simulink model "IDENTIFICACION_ARX_ARMAX"  (R2013a)
settings: Solver=ode5  SolverMode=SingleTasking  StartTime=0.0  StopTime=130  RelTol=1e-3
values from neighbouring files (symbols this model uses):
  lambda = 1    [generar_prbs.m]    (also in parametros_ident.m = 0.995)
undefined symbols (not defined in the file or in its folder): National_Instruments, PCI
libraries: rtwinlib x2
settings Model: SimulationMode=external  ExtModeTrigDuration=100000  Creator=n221  LastModifiedBy=u_labelectro
settings DataIOCC: SignalLoggingSaveFormat=ModelDataLogs
settings OptimizationCC: BlockReduction=off  BooleanDataType=off
settings DebuggingCC: SaveWithParameterizedLinksMsg=none  SignalResolutionControl=TryResolveAllWithWarning  SolverPrmCheckMsg=none  MultiTaskDSMMsg=warning  MultiTaskCondExecSysMsg=none  StrictBusMsg=None
settings HardwareCC: ProdIntDivRoundTo=Zero  ProdEndianess=LittleEndian  ProdHWDeviceType=Generic->32-bit x86 compatible  TargetIntDivRoundTo=Zero  TargetEndianess=LittleEndian  TargetHWDeviceType=MATLAB Host  ProdEqTarget=off
settings RTWCC: SystemTargetFile=rtwin.tlc  TemplateMakefile=rtwin.tmf  Description=Real-Time Windows Target  ProcessScript=rtwin_make_rtw_hook  IncludeERTFirstTime=on  RTWCompilerOptimization=On
settings CodeAppCC: MaxIdLength=95
settings RTWinTargetCC: TargetLibSuffix=_rtwin.lib  TargetPreCompLibLocation=D:\Real Time\toolbox\rtw\targets\rtwin\lib\win64  CodeReplacementLibrary=ANSI_C  RTWinDir=D:/REALTI~1/toolbox/rtw/targets/rtwin  TargetArch=win64

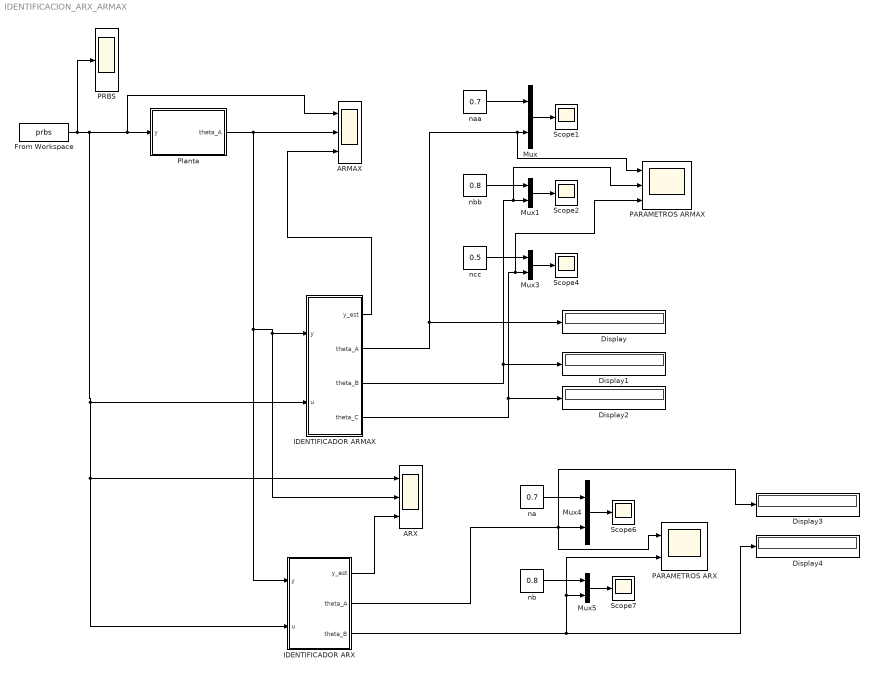
== system IDENTIFICACION_ARX_ARMAX ==
  ARMAX : Scope  NumInputPorts=3
      settings: TimeRange=130  YMin=20~42.5~45  YMax=20~70~75  SaveName=SALIDA_ARMAX  SampleInput=on  SampleTime=0.01
  ARX : Scope  NumInputPorts=3
      settings: YMin=-5~-5~-5  YMax=5~5~5  SaveName=SALIDA_ARX  SampleInput=on  SampleTime=0.01
  Display{,1..4} (5 alike) : Display
  From Workspace : FromWorkspace  VariableName=prbs  SampleTime=0.01
  IDENTIFICADOR ARMAX : Subsystem
  IDENTIFICADOR ARX : Subsystem
  Mux{,1,3..5} (5 alike) : Mux  Inputs=2
  PARAMETROS ARMAX : Scope  NumInputPorts=3
      settings: TimeRange=130  YMin=-0.99925~0.00075~0.005  YMax=-0.99475~0.00375~0.035  SaveName=PARAMETROS_ARMAX  SampleInput=on  SampleTime=0.01
  PARAMETROS ARX : Scope  NumInputPorts=2
      settings: TimeRange=600  YMin=-0.8~-5  YMax=0.8~5  SaveName=PARAMETROS_ARX  SampleInput=on  SampleTime=0.01
  PRBS : Scope
      settings: SaveName=ScopeData3  SampleInput=on  SampleTime=0.01
  Planta : Subsystem
  Scope{1..2,4,6..7} (5 alike) : Scope
      Scope1 settings: TimeRange=600  YMin=-0.8  YMax=0.8  SampleInput=on  SampleTime=0.01
      Scope2 settings: SaveName=ScopeData2  SampleInput=on  SampleTime=0.01
      Scope4 settings: SaveName=ScopeData4  SampleInput=on  SampleTime=0.01
      Scope6 settings: TimeRange=600  YMin=-0.8  YMax=0.8  SaveName=ScopeData6  SampleInput=on  SampleTime=0.01
      Scope7 settings: SaveName=ScopeData7  SampleInput=on  SampleTime=0.01
  na : Constant  Value=0.7
  "naa " : Constant  Value=0.7
  nb : Constant  Value=0.8
  nbb : Constant  Value=0.8
  ncc : Constant  Value=0.5
  wires:
  "naa "/1 -> Mux/1
  IDENTIFICADOR ARMAX/2(theta_A) -> PARAMETROS ARMAX/1, Mux/2, Display/1
  nbb/1 -> Mux1/1
  Mux1/1 -> Scope2/1
  Mux/1 -> Scope1/1
  IDENTIFICADOR ARMAX/3(theta_B) -> PARAMETROS ARMAX/2, Mux1/2, Display1/1
  IDENTIFICADOR ARMAX/4(theta_C) -> Display2/1, PARAMETROS ARMAX/3, Mux3/2
  Mux3/1 -> Scope4/1
  ncc/1 -> Mux3/1
  From Workspace/1 -> PRBS/1, ARX/1, IDENTIFICADOR ARX/2(u), IDENTIFICADOR ARMAX/2(u), Planta/1(y), ARMAX/1
  na/1 -> Mux4/1
  nb/1 -> Mux5/1
  Mux5/1 -> Scope7/1
  Mux4/1 -> Scope6/1
  IDENTIFICADOR ARX/2(theta_A) -> PARAMETROS ARX/1, Display3/1, Mux4/2
  IDENTIFICADOR ARX/3(theta_B) -> Display4/1, Mux5/2, PARAMETROS ARX/2
  IDENTIFICADOR ARMAX/1(y_est) -> ARMAX/3
  IDENTIFICADOR ARX/1(y_est) -> ARX/3
  Planta/1(theta_A) -> IDENTIFICADOR ARX/1(y), ARX/2, IDENTIFICADOR ARMAX/1(y), ARMAX/2

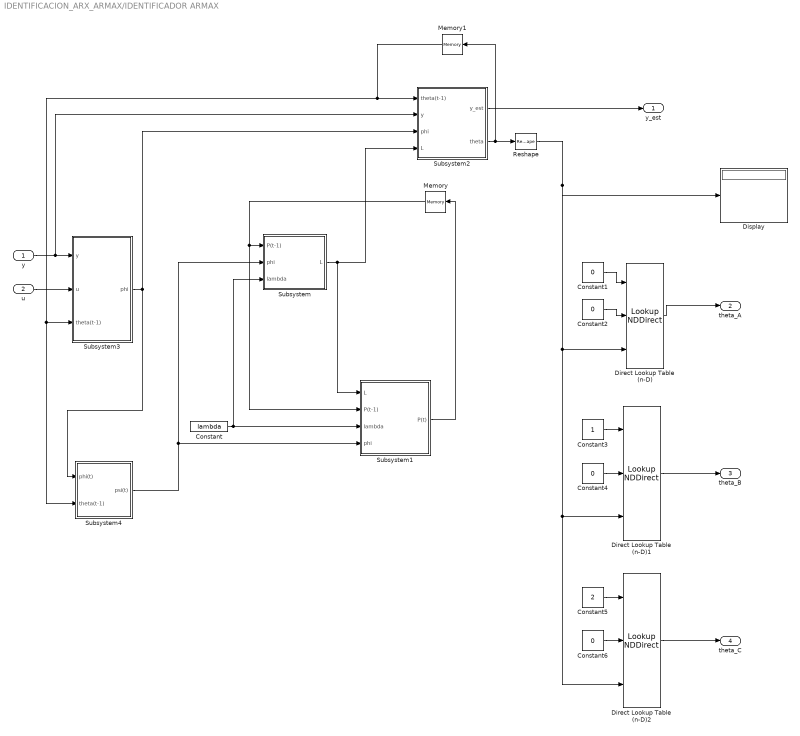
== system IDENTIFICACION_ARX_ARMAX/IDENTIFICADOR ARMAX ==
  y : Inport
  u : Inport  Port=2
  Constant : Constant  Value=lambda
  Constant{1..2,4,6} (4 alike) : Constant  Value=0
  Constant3 : Constant
  Constant5 : Constant  Value=2
  Direct Lookup Table (n-D) : LookupNDDirect  TableIsInput=on  Table=[4 5 ;16 19 ]  DiagnosticForOutOfRangeInput=Error  SampleTime=0.01
  Direct Lookup Table (n-D)1 : LookupNDDirect  TableIsInput=on  Table=[4 5 ;16 19 ]  DiagnosticForOutOfRangeInput=Error  SampleTime=0.01
  Direct Lookup Table (n-D)2 : LookupNDDirect  TableIsInput=on  Table=[4 5 ;16 19 ]  DiagnosticForOutOfRangeInput=Error  SampleTime=0.01
  Display : Display
  Memory : Memory  X0=1e6*eye(3)
  Memory1 : Memory
  Reshape : Reshape  OutputDimensionality=Column vector (2-D)
  Subsystem : Subsystem
  Subsystem1 : Subsystem
  Subsystem2 : Subsystem
  Subsystem3 : Subsystem
  Subsystem4 : Subsystem
  y_est : Outport
  theta_A : Outport  Port=2
  theta_B : Outport  Port=3
  theta_C : Outport  Port=4
  wires:
  y/1 -> Subsystem2/2(y), Subsystem3/1(y)
  Subsystem3/1(phi) -> Subsystem2/3(phi), Subsystem4/1(phi(t))
  Subsystem/1(L) -> Subsystem1/1(L), Subsystem2/4(L)
  u/1 -> Subsystem3/2(u)
  Constant/1 -> Subsystem1/3(lambda), Subsystem/3(lambda)
  Subsystem1/1(P(t)) -> Memory/1
  Memory/1 -> Subsystem1/2(P(t-1)), Subsystem/1(P(t-1))
  Subsystem2/1(y_est) -> y_est/1
  Subsystem2/2(theta) -> Reshape/1, Memory1/1
  Memory1/1 -> Subsystem4/2(theta(t-1)), Subsystem3/3(theta(t-1)), Subsystem2/1(theta(t-1))
  Constant4/1 -> Direct Lookup Table (n-D)1/2
  Constant3/1 -> Direct Lookup Table (n-D)1/1
  Constant1/1 -> Direct Lookup Table (n-D)/1
  Direct Lookup Table (n-D)/1 -> theta_A/1
  Direct Lookup Table (n-D)1/1 -> theta_B/1
  Constant2/1 -> Direct Lookup Table (n-D)/2
  Constant6/1 -> Direct Lookup Table (n-D)2/2
  Constant5/1 -> Direct Lookup Table (n-D)2/1
  Direct Lookup Table (n-D)2/1 -> theta_C/1
  Reshape/1 -> Direct Lookup Table (n-D)/3, Direct Lookup Table (n-D)2/3, Direct Lookup Table (n-D)1/3, Display/1
  Subsystem4/1(psi(t)) -> Subsystem1/4(phi), Subsystem/2(phi)

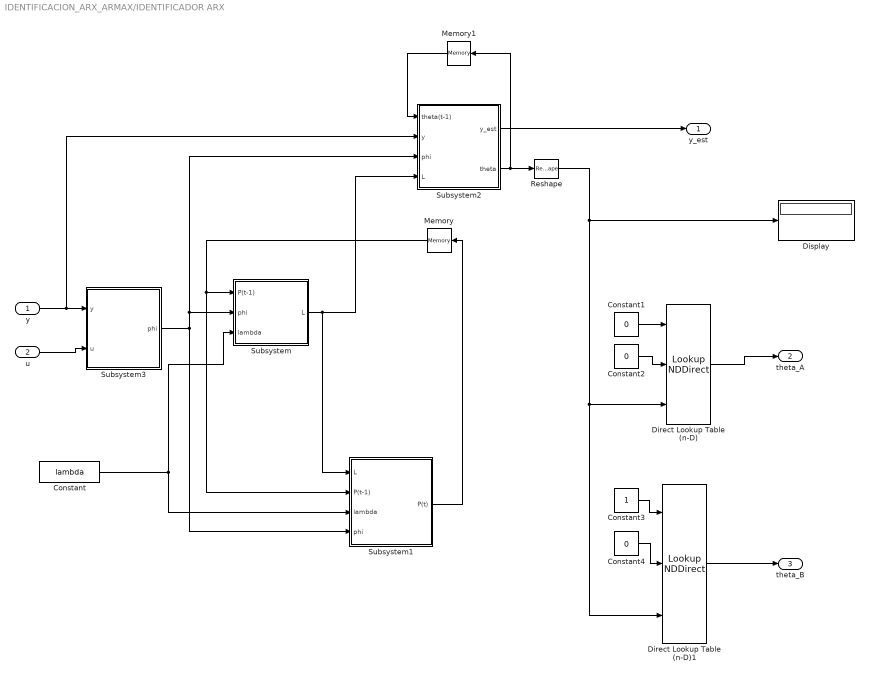
== system IDENTIFICACION_ARX_ARMAX/IDENTIFICADOR ARX ==
  y : Inport
  u : Inport  Port=2
  Constant : Constant  Value=lambda
  Constant1 : Constant  Value=0
  Constant2 : Constant  Value=0
  Constant3 : Constant
  Constant4 : Constant  Value=0
  Direct Lookup Table (n-D) : LookupNDDirect  TableIsInput=on  Table=[4 5 ;16 19 ]  DiagnosticForOutOfRangeInput=Error
  Direct Lookup Table (n-D)1 : LookupNDDirect  TableIsInput=on  Table=[4 5 ;16 19 ]  DiagnosticForOutOfRangeInput=Error
  Display : Display
  Memory : Memory  X0=1e6*eye(2)
  Memory1 : Memory
  Reshape : Reshape  OutputDimensionality=Column vector (2-D)
  Subsystem : Subsystem
  Subsystem1 : Subsystem
  Subsystem2 : Subsystem
  Subsystem3 : Subsystem
  y_est : Outport
  theta_A : Outport  Port=2
  theta_B : Outport  Port=3
  wires:
  y/1 -> Subsystem2/2(y), Subsystem3/1(y)
  Subsystem3/1(phi) -> Subsystem1/4(phi), Subsystem2/3(phi), Subsystem/2(phi)
  Subsystem/1(L) -> Subsystem1/1(L), Subsystem2/4(L)
  u/1 -> Subsystem3/2(u)
  Constant/1 -> Subsystem1/3(lambda), Subsystem/3(lambda)
  Subsystem1/1(P(t)) -> Memory/1
  Memory/1 -> Subsystem1/2(P(t-1)), Subsystem/1(P(t-1))
  Subsystem2/1(y_est) -> y_est/1
  Subsystem2/2(theta) -> Reshape/1, Memory1/1
  Memory1/1 -> Subsystem2/1(theta(t-1))
  Constant4/1 -> Direct Lookup Table (n-D)1/2
  Constant3/1 -> Direct Lookup Table (n-D)1/1
  Constant2/1 -> Direct Lookup Table (n-D)/2
  Constant1/1 -> Direct Lookup Table (n-D)/1
  Reshape/1 -> Direct Lookup Table (n-D)1/3, Direct Lookup Table (n-D)/3, Display/1
  Direct Lookup Table (n-D)/1 -> theta_A/1
  Direct Lookup Table (n-D)1/1 -> theta_B/1

== system IDENTIFICACION_ARX_ARMAX/Planta ==
  y : Inport
  Analog Input : rtwinlib/Analog Input  SampleTime=0.1  MaxMissedTicks=10  ShowMissedTicks=off  YieldWhenWaiting=off  DrvName=National_Instruments/PCI-6229  DrvAddress=4294967295  DrvOptions=[0 0 0 0 0]  Channels=1  RangeMode=1  VoltRange=1  DataType=1
      settings: AttributesFormatString=National Instruments\nPCI-6229 [auto]
  Analog Output : rtwinlib/Analog Output  SampleTime=0.1  MaxMissedTicks=10  ShowMissedTicks=off  YieldWhenWaiting=off  DrvName=National_Instruments/PCI-6229  DrvAddress=4294967295  DrvOptions=[0 0 0 0 0]  Channels=1  RangeMode=1  VoltRange=1  InitialValue=[]  FinalValue=[]
      settings: AttributesFormatString=National Instruments\nPCI-6229 [auto]
  Fcn : Fcn  Expr=0.2*u(1)-10
  Fcn1 : Fcn  Expr=25*u(1)-25
  theta_A : Outport
  wires:
  Fcn/1 -> Analog Output/1
  y/1 -> Fcn/1
  Analog Input/1 -> Fcn1/1
  Fcn1/1 -> theta_A/1

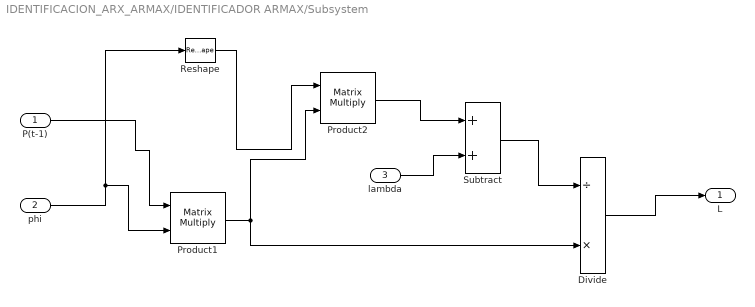
== system IDENTIFICACION_ARX_ARMAX/IDENTIFICADOR ARMAX/Subsystem ==
  P(t-1) : Inport
  phi : Inport  Port=2
  lambda : Inport  Port=3
  Divide : Product  Inputs=/*
  Product1 : Product  Multiplication=Matrix(*)  SampleTime=0.01
  Product2 : Product  Multiplication=Matrix(*)  SampleTime=0.01
  Reshape : Reshape  OutputDimensionality=Row vector (2-D)
  Subtract : Sum
  L : Outport
  wires:
  Divide/1 -> L/1
  Subtract/1 -> Divide/1
  phi/1 -> Product1/2, Reshape/1
  Reshape/1 -> Product2/1
  lambda/1 -> Subtract/2
  Product1/1 -> Divide/2, Product2/2
  P(t-1)/1 -> Product1/1
  Product2/1 -> Subtract/1

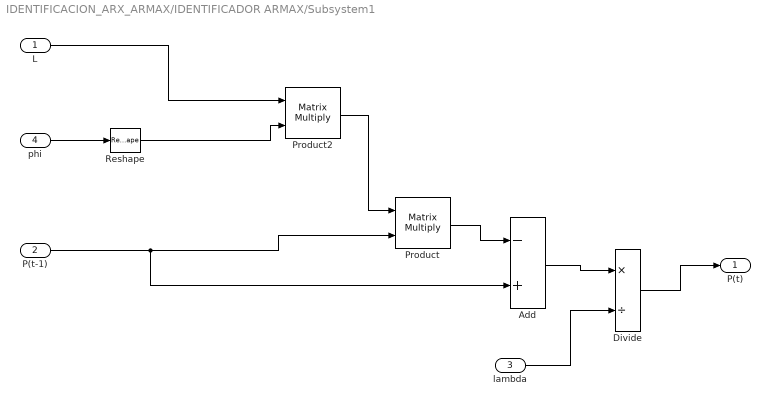
== system IDENTIFICACION_ARX_ARMAX/IDENTIFICADOR ARMAX/Subsystem1 ==
  L : Inport
  P(t-1) : Inport  Port=2
  lambda : Inport  Port=3
  phi : Inport  Port=4
  Add : Sum  Inputs=-+
  Divide : Product  Inputs=*/
  Product : Product  Multiplication=Matrix(*)  SampleTime=0.01
  Product2 : Product  Multiplication=Matrix(*)  SampleTime=0.01
  Reshape : Reshape  OutputDimensionality=Row vector (2-D)
  P(t) : Outport
  wires:
  L/1 -> Product2/1
  phi/1 -> Reshape/1
  Reshape/1 -> Product2/2
  Product2/1 -> Product/1
  P(t-1)/1 -> Product/2, Add/2
  Product/1 -> Add/1
  Add/1 -> Divide/1
  Divide/1 -> P(t)/1
  lambda/1 -> Divide/2

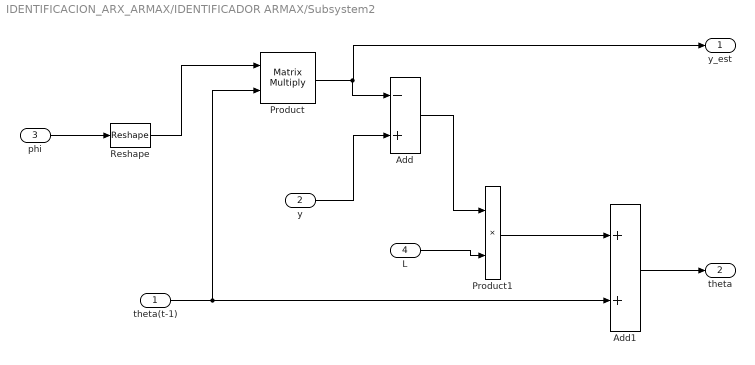
== system IDENTIFICACION_ARX_ARMAX/IDENTIFICADOR ARMAX/Subsystem2 ==
  theta(t-1) : Inport
  y : Inport  Port=2
  phi : Inport  Port=3
  L : Inport  Port=4
  Add : Sum  Inputs=-+
  Add1 : Sum
  Product : Product  Multiplication=Matrix(*)  SampleTime=0.01
  Product1 : Product
  Reshape : Reshape  OutputDimensionality=Row vector (2-D)
  y_est : Outport
  theta : Outport  Port=2
  wires:
  Product/1 -> Add/1, y_est/1
  y/1 -> Add/2
  L/1 -> Product1/2
  Add/1 -> Product1/1
  Product1/1 -> Add1/1
  Add1/1 -> theta/1
  theta(t-1)/1 -> Product/2, Add1/2
  Reshape/1 -> Product/1
  phi/1 -> Reshape/1

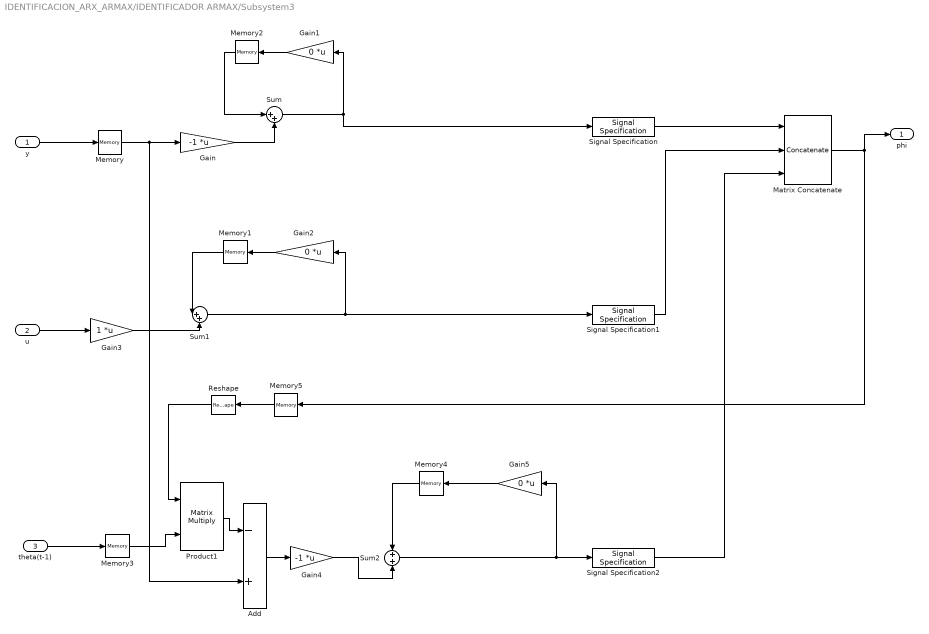
== system IDENTIFICACION_ARX_ARMAX/IDENTIFICADOR ARMAX/Subsystem3 ==
  y : Inport
  u : Inport  Port=2
  theta(t-1) : Inport  Port=3
  Add : Sum  Inputs=-+
  Gain : Gain  Gain=-1  Multiplication=Matrix(K*u)
  Gain1 : Gain  Gain=0  Multiplication=Matrix(K*u)
  Gain2 : Gain  Gain=0  Multiplication=Matrix(K*u)
  Gain3 : Gain  Multiplication=Matrix(K*u)
  Gain4 : Gain  Gain=-1  Multiplication=Matrix(K*u)
  Gain5 : Gain  Gain=0  Multiplication=Matrix(K*u)
  Matrix Concatenate : Concatenate  NumInputs=3  Mode=Multidimensional array
  Memory{,1..5} (6 alike) : Memory
  Product1 : Product  Multiplication=Matrix(*)  SampleTime=0.01
  Reshape : Reshape  OutputDimensionality=Row vector (2-D)
  Signal Specification : SignalSpecification  Dimensions=[1 1]
  Signal Specification1 : SignalSpecification  Dimensions=[1 1]
  Signal Specification2 : SignalSpecification  Dimensions=[1 1]
  Sum : Sum  Inputs=|++
  Sum1 : Sum  Inputs=|++
  Sum2 : Sum
  phi : Outport
  wires:
  Sum/1 -> Gain1/1, Signal Specification/1
  Gain1/1 -> Memory2/1
  Memory2/1 -> Sum/1
  Gain/1 -> Sum/2
  Memory/1 -> Add/2, Gain/1
  y/1 -> Memory/1
  Gain2/1 -> Memory1/1
  u/1 -> Gain3/1
  Gain3/1 -> Sum1/2
  Memory1/1 -> Sum1/1
  Sum1/1 -> Gain2/1, Signal Specification1/1
  Signal Specification/1 -> Matrix Concatenate/1
  Signal Specification1/1 -> Matrix Concatenate/2
  Matrix Concatenate/1 -> phi/1, Memory5/1
  theta(t-1)/1 -> Memory3/1
  Reshape/1 -> Product1/1
  Memory5/1 -> Reshape/1
  Memory3/1 -> Product1/2
  Add/1 -> Gain4/1
  Gain4/1 -> Sum2/2
  Memory4/1 -> Sum2/1
  Gain5/1 -> Memory4/1
  Sum2/1 -> Gain5/1, Signal Specification2/1
  Signal Specification2/1 -> Matrix Concatenate/3
  Product1/1 -> Add/1

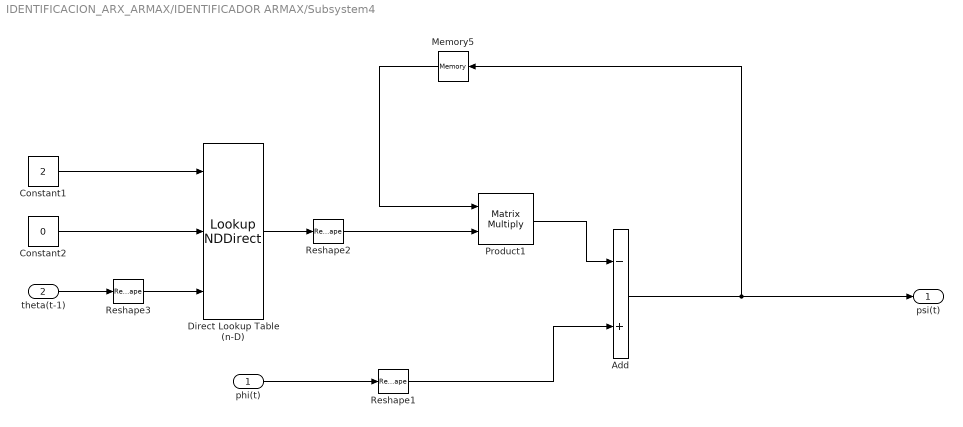
== system IDENTIFICACION_ARX_ARMAX/IDENTIFICADOR ARMAX/Subsystem4 ==
  phi(t) : Inport
  theta(t-1) : Inport  Port=2
  Add : Sum  Inputs=-+
  Constant1 : Constant  Value=2
  Constant2 : Constant  Value=0
  Direct Lookup Table (n-D) : LookupNDDirect  TableIsInput=on  Table=[4 5 ;16 19 ]  DiagnosticForOutOfRangeInput=Error  SampleTime=0.01
  Memory5 : Memory
  Product1 : Product  Multiplication=Matrix(*)  SampleTime=0.01
  Reshape1 : Reshape  OutputDimensionality=Column vector (2-D)
  Reshape2 : Reshape  OutputDimensionality=Column vector (2-D)
  Reshape3 : Reshape  OutputDimensionality=Column vector (2-D)
  psi(t) : Outport
  wires:
  Memory5/1 -> Product1/1
  Add/1 -> Memory5/1, psi(t)/1
  phi(t)/1 -> Reshape1/1
  Reshape1/1 -> Add/2
  Reshape2/1 -> Product1/2
  theta(t-1)/1 -> Reshape3/1
  Constant1/1 -> Direct Lookup Table (n-D)/1
  Constant2/1 -> Direct Lookup Table (n-D)/2
  Direct Lookup Table (n-D)/1 -> Reshape2/1
  Reshape3/1 -> Direct Lookup Table (n-D)/3
  Product1/1 -> Add/1

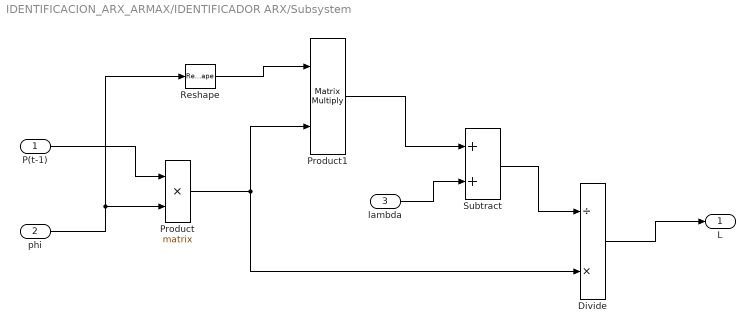
== system IDENTIFICACION_ARX_ARMAX/IDENTIFICADOR ARX/Subsystem ==
  P(t-1) : Inport
  phi : Inport  Port=2
  lambda : Inport  Port=3
  Divide : Product  Inputs=/*
  Product : Product  Multiplication=Matrix(*)
  Product1 : Product  Multiplication=Matrix(*)
  Reshape : Reshape  OutputDimensionality=Row vector (2-D)
  Subtract : Sum
  L : Outport
  wires:
  Divide/1 -> L/1
  Subtract/1 -> Divide/1
  phi/1 -> Reshape/1, Product/2
  Reshape/1 -> Product1/1
  Product1/1 -> Subtract/1
  lambda/1 -> Subtract/2
  Product/1 -> Product1/2, Divide/2
  P(t-1)/1 -> Product/1

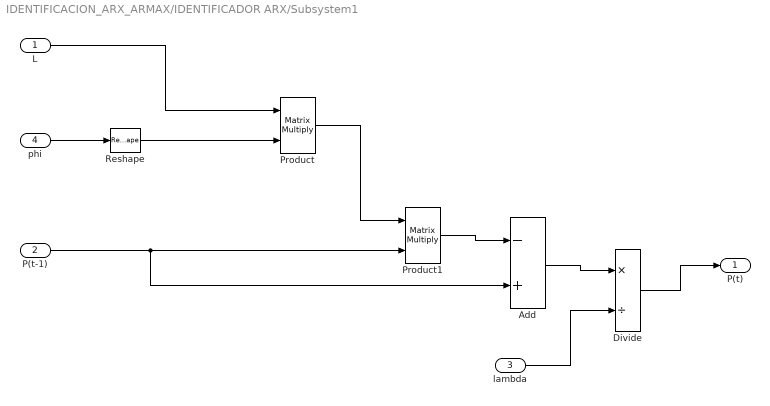
== system IDENTIFICACION_ARX_ARMAX/IDENTIFICADOR ARX/Subsystem1 ==
  L : Inport
  P(t-1) : Inport  Port=2
  lambda : Inport  Port=3
  phi : Inport  Port=4
  Add : Sum  Inputs=-+
  Divide : Product  Inputs=*/
  Product : Product  Multiplication=Matrix(*)
  Product1 : Product  Multiplication=Matrix(*)
  Reshape : Reshape  OutputDimensionality=Row vector (2-D)
  P(t) : Outport
  wires:
  L/1 -> Product/1
  phi/1 -> Reshape/1
  Reshape/1 -> Product/2
  Product/1 -> Product1/1
  P(t-1)/1 -> Add/2, Product1/2
  Product1/1 -> Add/1
  Add/1 -> Divide/1
  Divide/1 -> P(t)/1
  lambda/1 -> Divide/2

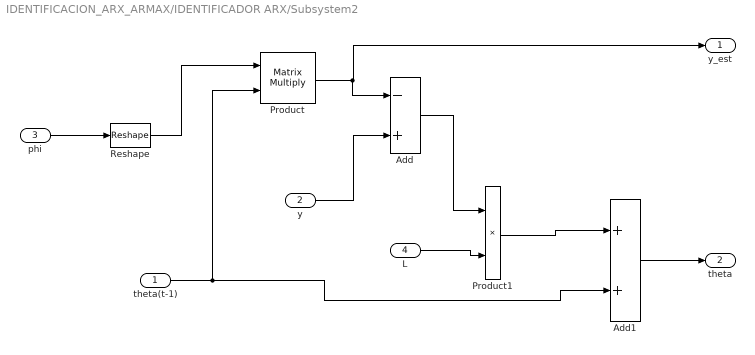
== system IDENTIFICACION_ARX_ARMAX/IDENTIFICADOR ARX/Subsystem2 ==
  theta(t-1) : Inport
  y : Inport  Port=2
  phi : Inport  Port=3
  L : Inport  Port=4
  Add : Sum  Inputs=-+
  Add1 : Sum
  Product : Product  Multiplication=Matrix(*)
  Product1 : Product
  Reshape : Reshape  OutputDimensionality=Row vector (2-D)
  y_est : Outport
  theta : Outport  Port=2
  wires:
  Product/1 -> Add/1, y_est/1
  y/1 -> Add/2
  L/1 -> Product1/2
  Add/1 -> Product1/1
  Product1/1 -> Add1/1
  Add1/1 -> theta/1
  theta(t-1)/1 -> Product/2, Add1/2
  Reshape/1 -> Product/1
  phi/1 -> Reshape/1

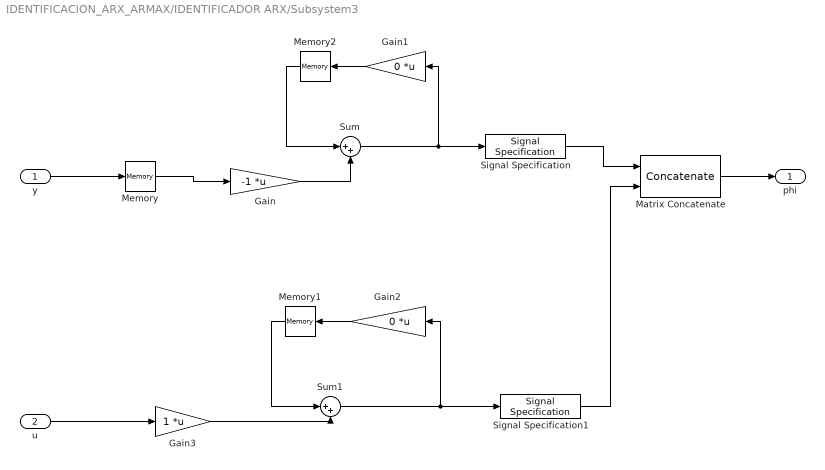
== system IDENTIFICACION_ARX_ARMAX/IDENTIFICADOR ARX/Subsystem3 ==
  y : Inport
  u : Inport  Port=2
  Gain : Gain  Gain=-1  Multiplication=Matrix(K*u)
  Gain1 : Gain  Gain=0  Multiplication=Matrix(K*u)
  Gain2 : Gain  Gain=0  Multiplication=Matrix(K*u)
  Gain3 : Gain  Multiplication=Matrix(K*u)
  Matrix Concatenate : Concatenate  Mode=Multidimensional array
  Memory : Memory
  Memory1 : Memory
  Memory2 : Memory
  Signal Specification : SignalSpecification  Dimensions=[1 1]
  Signal Specification1 : SignalSpecification  Dimensions=[1 1]
  Sum : Sum  Inputs=|++
  Sum1 : Sum  Inputs=|++
  phi : Outport
  wires:
  Sum/1 -> Gain1/1, Signal Specification/1
  Gain1/1 -> Memory2/1
  Memory2/1 -> Sum/1
  Gain/1 -> Sum/2
  Memory/1 -> Gain/1
  y/1 -> Memory/1
  Gain2/1 -> Memory1/1
  u/1 -> Gain3/1
  Gain3/1 -> Sum1/2
  Memory1/1 -> Sum1/1
  Sum1/1 -> Signal Specification1/1, Gain2/1
  Signal Specification/1 -> Matrix Concatenate/1
  Signal Specification1/1 -> Matrix Concatenate/2
  Matrix Concatenate/1 -> phi/1
